simulink model "zad2_rep_gr"  (R2016b)
settings: Solver=VariableStepAuto  StartTime=0.0  StopTime=10.0  RelTol=1e-3
undefined symbols (not defined in the file or in its folder): Tp
settings Model: Creator=tomasz  LastModifiedBy=tomasz

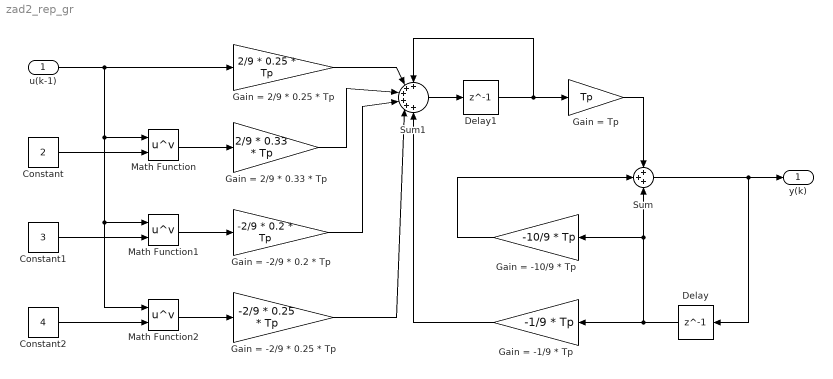
== system zad2_rep_gr ==
  u(k-1) : Inport
  Constant : Constant  Value=2
  Constant1 : Constant  Value=3
  Constant2 : Constant  Value=4
  Delay : Delay  DelayLength=1  InitialCondition=0
  Delay1 : Delay  DelayLength=1  InitialCondition=0
  Gain = -1/9 * Tp : Gain  Gain=-1/9 * Tp
  Gain = -10/9 * Tp : Gain  Gain=-10/9 * Tp
  Gain = -2/9 * 0.2 * Tp : Gain  Gain=-2/9 * 0.2 * Tp
  Gain = -2/9 * 0.25 * Tp : Gain  Gain=-2/9 * 0.25 * Tp
  Gain = 2/9 * 0.25 * Tp : Gain  Gain=2/9 * 0.25 * Tp
  Gain = 2/9 * 0.33 * Tp : Gain  Gain=2/9 * 0.33 * Tp
  Gain = Tp : Gain  Gain=Tp
  Math Function : Math  Operator=pow  SaturateOnIntegerOverflow=on
  Math Function1 : Math  Operator=pow  SaturateOnIntegerOverflow=on
  Math Function2 : Math  Operator=pow  SaturateOnIntegerOverflow=on
  Sum : Sum  Inputs=+++
  Sum1 : Sum  Inputs=++++++
  y(k) : Outport
  wires:
  Delay/1 -> Sum/3, Gain = -10/9 * Tp/1, Gain = -1/9 * Tp/1
  Sum/1 -> y(k)/1, Delay/1
  Gain = -10/9 * Tp/1 -> Sum/2
  Sum1/1 -> Delay1/1
  Delay1/1 -> Sum1/1, Gain = Tp/1
  Gain = Tp/1 -> Sum/1
  Gain = -1/9 * Tp/1 -> Sum1/6
  Constant2/1 -> Math Function2/2
  Constant1/1 -> Math Function1/2
  Constant/1 -> Math Function/2
  u(k-1)/1 -> Math Function2/1, Math Function1/1, Math Function/1, Gain = 2/9 * 0.25 * Tp/1
  Gain = 2/9 * 0.25 * Tp/1 -> Sum1/2
  Math Function/1 -> Gain = 2/9 * 0.33 * Tp/1
  Gain = 2/9 * 0.33 * Tp/1 -> Sum1/3
  Math Function2/1 -> Gain = -2/9 * 0.25 * Tp/1
  Math Function1/1 -> Gain = -2/9 * 0.2 * Tp/1
  Gain = -2/9 * 0.2 * Tp/1 -> Sum1/4
  Gain = -2/9 * 0.25 * Tp/1 -> Sum1/5
